simulink model "damiao"  (R2022b)
settings: Solver=VariableStepAuto  StartTime=0.0  StopTime=inf  RelTol=1e-3
libraries: simulink x4, RTBoxbasiclib x1, etargetslib x1
settings Model: Creator=admin  LastModifiedBy=admin

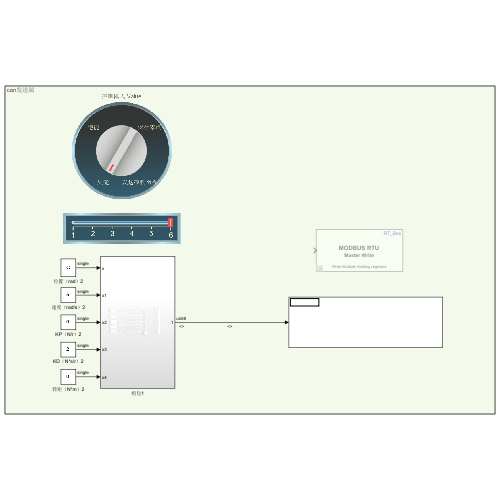
[thumbnail: Simulink's stored preview of the top-level diagram]
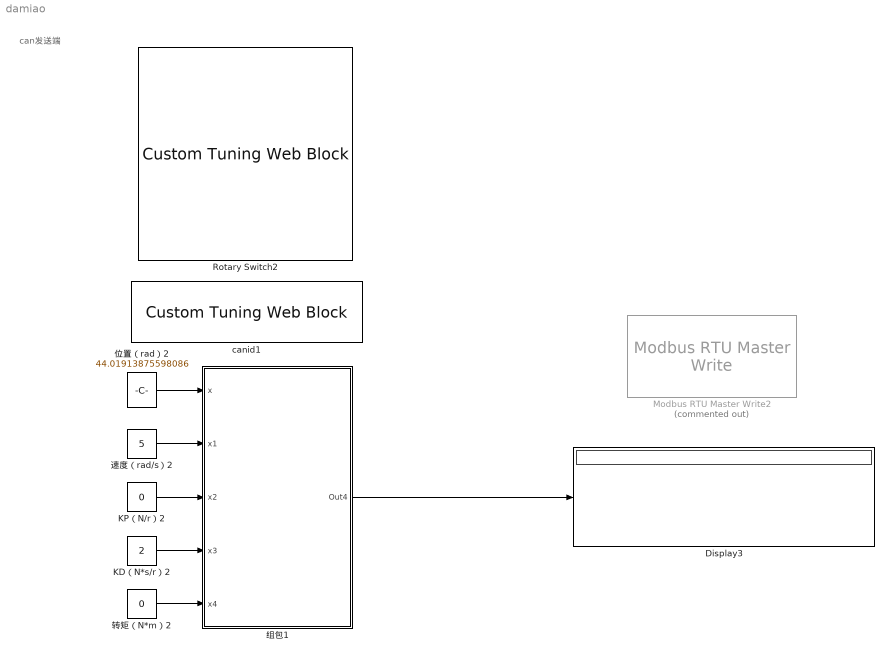
== system damiao ==
  note: can发送端
  Display3 : Display
      settings: Format=hex (Stored Integer)
  KD（N*s/r）2 : Constant  Value=2  OutDataTypeStr=single
  KP（N/r）2 : Constant  Value=0  OutDataTypeStr=single
  Modbus RTU Master Write2 : RTBoxbasiclib/Modbus RTU Master Write  Commented=on  Server_Port=/dev/ttyUSB0  Function=Write Multiple Holding registers  CoilAddress=0  HoldingRegisterAddress=0  numElements_coil=1  numElements_holdingReg=8  SampleTime=0.1  Slave_ID=1  Baudrate=1000  parity_=N  data_bit=8  stop_bit=1  responese_to_sec=0  responese_to_usec=0
      settings: SourceProductName=RT Box Simulink support
  Rotary Switch2 : CustomTuningWebBlock  ShowInitialText=on  Configuration="{\"type\":\"RotarySwitch\",\"settings\":{\"BindingType\":\"param\",\"backgroundColor\":[0,0,255,\"1\"],\"backgroundOffset\":1,\"fixedAspectRatio\":\"on\",\"image\":{\"size\":[150,150],\"src\":\"data:image/svg+xml;base64,PD94bWwgdmVyc2lvbj0iMS4wIiBlbmNvZGluZz0iVVRGLTgiIHN0YW5kYWxvbmU9Im5vIj8+CjwhLS0gR2VuZXJhdG9yOiBBZG9iZSBJbGx1c3RyYXRvciAxOS4yLjEsIFNWRyBFeHBvcnQgUGx1Zy1JbiAuIFNWRyBWZXJzaW9uOiA2LjAwIEJ1aWxkIDApICAtLT4KCjxzdmcKICAgeG1sbnM6ZGM9Imh0dHA6Ly9wdXJsLm9yZy9kYy9lbGVtZW50cy8xLjEvIgogICB4bWxuczpjYz0iaHR0cDovL2NyZWF0aXZlY29tbW9ucy5vcmcvbnMjIgogICB4bWxuczpyZGY9Imh0dHA6Ly93d3cudzMub3JnLzE5OTkvMDIvMjItcmRmLXN5bnRh ...(+9660 chars)\"},\"showBackgroundColor\":false,\"variant\":\"rotarySwitch\"},\"components\":[{\"name\":\"RotarySwitchComponent\",\"settings\":{\"arcAngle\":300,\"arcAngleOffset\":120,\"handle\":{\"size\":[150,150],\"src\":\"data:image/svg+xml;base64,PHN2ZyBpZD0iTGF5ZXJfMSIgZGF0YS1uYW1lPSJMYXllciAxIiB4bWxucz0iaHR0cDovL3d3dy53My5vcmcvMjAwMC9zdmciIHhtbG5zOnhsaW5rPSJodHRwOi8vd3d3LnczLm9yZy8xOTk5L3hsaW5rIiB2aWV3Qm94PSIwIDAgMTIxIDEyMSI+PGRlZnM+PHN0eWxlPi5jbHMtMXtmaWxsOnVybCgjbGluZWFyLWdyYWRpZW50KTt9LmNscy0yLC5jbHMtM3tmaWxsOiNkMWQxZDE7fS5jbHMtM3tzdHJva2U6I2I3YjdiNztzdHJva2UtbWl0ZXJsaW1pdDoxMDtzdHJva2Utd2lkdGg6MC4yNXB4O30uY2xzLTR7ZmlsbDojZjMwMDAwO30uY2xzLTV7ZmlsbDojZjIxNzY3O308L3N0eWxlPjxsaW5lYXJHcmFkaWVudCBpZD0ibGluZWFyLWdyYWRpZW50IiB4MT0iNjAuNSIgeTE9IjEyMC41IiB4Mj0iNjAuNSIgeTI9IjAuNSIgZ3JhZGllbnRVbml0cz0idXNlclNwYWNlT25Vc2UiPjxzdG9wIG9mZnNldD0iMCIgc3RvcC1jb2xvcj0iI2QxZDFkMSIvPjxzdG9wIG9mZnNldD0iMC4xIiBzdG9wLWNvbG9yPSIjY2VjZWNlIi8+PHN0b3Agb2Zmc2V0PSIwLjE5IiBzdG9wLWNvbG9yPSIjYzNjM2MzIi8+PHN0b3Agb2Zmc2V0PSIwLjI4IiBzdG9wLWNvbG9yPSIjYjFiMWIxIi8+PHN0b3Agb2Zmc2V0PSIwLjM2IiBzdG9wLWNvbG9yPSIjOTg5ODk4Ii8+PHN0b3Agb2Zmc2V0PSIwLjQ0IiBzdG9wLWNvbG9yPSIjNzg3ODc4Ii8+PHN0b3Agb2Zmc2V0PSIwLjQ2IiBzdG9wLWNvbG9yPSIjNmI2YjZiIi8+PHN0b3Agb2Zmc2V0PSIwLjU0IiBzdG9wLWNvbG9yPSIjNmI2YjZiIi8+PHN0b3Agb2Zmc2V0PSIwLjU2IiBzdG9wLWNvbG9yPSIjNzY3Njc2Ii8+PHN0b3Agb2Zmc2V0PSIwLjY0IiBzdG9wLWNvbG9yPSIjOTc5Nzk3Ii8+PHN0b3Agb2Zmc2V0PSIwLjcyIiBzdG9wLWNvbG9yPSIjYjBiMGIwIi8+PHN0b3Agb2Zmc2V0PSIwLjgxIiBzdG9wLWNvbG9yPSIjYzNjM2MzIi8+PHN0b3Agb2Zmc2V0PSIwLjkiIHN0b3AtY29sb3I9IiNjZGNkY2QiLz48c3RvcCBvZmZzZXQ9IjEiIHN0b3AtY29sb3I9IiNkMWQxZDEiLz48L2xpbmVhckdyYWRpZW50PjwvZGVmcz48Y2lyY2xlIGNsYXNzPSJjbHMtMSIgY3g9IjYwLjUiIGN5PSI2MC41IiByPSI2MCIvPjxwYXRoIGNsYXNzPSJjbHMtMiIgZD0iTTYwLjUsMUE1OS41LDU5LjUsMCwxLDEsMSw2MC41LDU5LjU3LDU5LjU3LDAsMCwxLDYwLjUsMW0wLTFBNjAuNSw2MC41LDAsMSwwLDEyMSw2MC41LDYwLjUsNjAuNSwwLDAsMCw2MC41LDBaIi8+PHJlY3QgY2xhc3M9ImNscy0zIiB4PSIwLjUiIHk9IjUxLjUiIHdpZHRoPSIxMjAiIGhlaWdodD0iMTgiIHJ4PSIzLjA0Ii8+PHJlY3QgY2xhc3M9ImNscy00IiB4PSI1Ljc1IiB5PSI1OC43NSIgd2lkdGg9IjE2IiBoZWlnaHQ9IjMiLz48cGF0aCBjbGFzcz0iY2xzLTUiIGQ9Ik0yMS4yNSw1OS4yNXYyaC0xNXYtMmgxNW0xLTFoLTE3djRoMTd2LTRaIi8+PC9zdmc+\"},\"handleOffset\":[0,0],\"handleOrientation\":180,\"handlePosition\":[0,0,1,1],\"handleSize\":{\"height\":0.5,\"width\":0.5},\"labelRadius\":0.36,\"position\":[0,0,1,1],\"states\":[{\"Label\":{\"color\":[0,0,0,1],\"icon\":{\"size\":[0,0],\"src\":[],\"srcOrientation\":\"Right\"},\"iconPlacement\":\"left\",\"opacity\":1,\"position\":[0.7345552884615385,0.6796274038461538],\"show\":true,\"text\":{\"content\":\"失能\",\"font\":\"Helvetica\",\"fontSize\":24}},\"Value\":0},{\"Label\":{\"color\":[0,0,0,1],\"icon\":{\"size\":[0,0],\"src\":[],\"srcOrientation\":\"Right\"},\"iconPlacement\":\"left\",\"opacity\":1,\"position\":[0.35757211538461536,0.7603966346153846],\"show\":true,\"text\":{\"content\":\"使能\",\"font\":\"Helvetica\",\"fontSize\":24}},\"Value\":1},{\"Label\":{\"color\":[0,0,0,1],\"icon\":{\"size\":[0,0],\"src\":[],\"srcOrientation\":\"Right\"},\"iconPlacement\":\"left\",\"opacity\":1,\"position\":[0.09603365384615385,0.46033653846153844],\"show\":true,\"text\":{\"content\":\"保存零点\",\"font\":\"Helvetica\",\"fontSize\":24}},\"Value\":2},{\"Label\":{\"color\":[0,0,0,1],\"icon\":{\"size\":[0,0],\"src\":[],\"srcOrientation\":\"Right\"},\"iconPlacement\":\"left\",\"opacity\":1,\"position\":[0.36532451923076925,0.1180889423076923],\"show\":true,\"text\":{\"content\":\"发送控制命令\",\"font\":\"Helvetica\",\"fontSize\":24}},\"Value\":3}],\"tickRadius\":0.32}},{\"name\":\"BackgroundImageComponent\",\"settings\":{\"image\":{\"size\":[155,150],\"src\":\"data:image/svg+xml;base64,PD94bWwgdmVyc2lvbj0iMS4wIiBlbmNvZGluZz0idXRmLTgiPz4NCjwhLS0gR2VuZXJhdG9yOiBBZG9iZSBJbGx1c3RyYXRvciAyNS4wLjAsIFNWRyBFeHBvcnQgUGx1Zy1JbiAuIFNWRyBWZXJzaW9uOiA2LjAwIEJ1aWxkIDApICAtLT4NCjxzdmcgdmVyc2lvbj0iMS4xIg0KCSBpZD0iTGF5ZXJfMl8xXyIgeG1sbnM6Y2M9Imh0dHA6Ly9jcmVhdGl2ZWNvbW1vbnMub3JnL25zIyIgeG1sbnM6ZGM9Imh0dHA6Ly9wdXJsLm9yZy9kYy9lbGVtZW50cy8xLjEvIiB4bWxuczppbmtzY2FwZT0iaHR0cDovL3d3dy5pbmtzY2FwZS5vcmcv ...(+4184 chars)\",\"srcOrientation\":\"Right\"},\"position\":[0,0,1,1],\"scaleMode\":\"0\"}},{\"name\":\"ForegroundImageComponent\",\"settings\":{\"image\":{\"size\":[0,0],\"src\":\"default\",\"srcOrientation\":[]},\"isForeground\":1,\"position\":[0,0,1,1],\"scaleMode\":\"0\"}}]}"
  canid1 : CustomTuningWebBlock  LabelPosition=Hide  ShowInitialText=on  Configuration="{\"type\":\"LinearGauge\",\"settings\":{\"BindingType\":\"param\",\"aspectRatio\":3.7777777777777777,\"backgroundColor\":[0,0,0,\"1\"],\"backgroundOffset\":0,\"backgroundOpacity\":1,\"fixedAspectRatio\":\"on\",\"foregroundColor\":[252,252,196],\"orientation\":\"horizontal\",\"showBackgroundColor\":false,\"value\":0},\"components\":[{\"name\":\"LinearScaleComponent\",\"settings\":{\"bounds\":{\"max\":6,\"min\":1,\"tickInterval\":1},\"internalTickHeightScaleFactor\":0.5,\"labelColor\":[255,255,200],\"labelFont\":{\"font\":\"Arial\",\"fontSize\":12},\"labelOffset\":0.05,\"labelTransparency\":1,\"needleImage\":{\"size\":[596,842],\"src\":\"data:image/svg+xml;base64,PD94bWwgdmVyc2lvbj0iMS4wIiBlbmNvZGluZz0idXRmLTgiPz4NCjwhLS0gR2VuZXJhdG9yOiBBZG9iZSBJbGx1c3RyYXRvciAyNS4wLjAsIFNWRyBFeHBvcnQgUGx1Zy1JbiAuIFNWRyBWZXJzaW9uOiA2LjAwIEJ1aWxkIDApICAtLT4NCjxzdmcgdmVyc2lvbj0iMS4xIg0KCSBpZD0ic3ZnOCIgeG1sbnM6Y2M9Imh0dHA6Ly9jcmVhdGl2ZWNvbW1vbnMub3JnL25zIyIgeG1sbnM6ZGM9Imh0dHA6Ly9wdXJsLm9yZy9kYy9lbGVtZW50cy8xLjEvIiB4bWxuczppbmtzY2FwZT0iaHR0cDovL3d3dy5pbmtzY2FwZS5vcmcvbmFtZXNw ...(+2420 chars)\",\"srcOrientation\":\"Right\"},\"needleOffset\":[-0.8044596912521441,-0.0642123287671233],\"needleSize\":{\"height\":0.4337797619047619,\"width\":0.07668067226890757},\"position\":[0.2829861111111111,0.04398634453781513,0.9196428571428571,0.6088789682539683],\"referencePoint\":\"auto\",\"scaleColors\":[],\"scaleColorsSize\":0.2,\"scaleDirection\":\"LR\",\"showLabels\":1,\"showMinorTicks\":0,\"showSpanLine\":1,\"showTicks\":1,\"tickColor\":[252,252,197],\"tickTransparency\":1,\"valueBarColor\":[0,114,189],\"valueBarOffset\":-0.27,\"valueBarSize\":0.1,\"valueBarTransparency\":1}},{\"name\":\"BackgroundImageComponent\",\"settings\":{\"image\":{\"size\":[380,101],\"src\":\"data:image/svg+xml;base64,PHN2ZyB4bWxucz0iaHR0cDovL3d3dy53My5vcmcvMjAwMC9zdmciIHhtbG5zOnhsaW5rPSJodHRwOi8vd3d3LnczLm9yZy8xOTk5L3hsaW5rIiB2aWV3Qm94PSIwIDAgMzgwIDEwMSI+PGRlZnM+PHN0eWxlPi5jbHMtMXtmaWxsOiMwMDJiNDI7fS5jbHMtMntmaWxsOiM0MjcwODI7fS5jbHMtM3tmaWxsOnVybCgjcmFkaWFsLWdyYWRpZW50KTt9LmNscy00e2ZpbGw6I2M4YzhjODtzdHJva2U6IzAwMDt9PC9zdHlsZT48cmFkaWFsR3JhZGllbnQgaWQ9InJhZGlhbC1ncmFkaWVudCIgY3g9IjE5MCIgY3k9IjUwLjUiIHI9IjI2OS4yMSIgZ3JhZGllbnRVbml0cz0idXNlclNwYWNlT25Vc2UiPjxzdG9wIG9mZnNldD0iMC4wMSIgc3RvcC1jb2xvcj0iIzNlNGY1OCIvPjxzdG9wIG9mZnNldD0iMC4wNiIgc3RvcC1jb2xvcj0iIzQ0NTc2MSIvPjxzdG9wIG9mZnNldD0iMC4xNSIgc3RvcC1jb2xvcj0iIzU1NmE3NiIvPjxzdG9wIG9mZnNldD0iMC4yNSIgc3RvcC1jb2xvcj0iIzZkODg5NSIvPjxzdG9wIG9mZnNldD0iMC4zOCIgc3RvcC1jb2xvcj0iIzhmYjJjMyIvPjxzdG9wIG9mZnNldD0iMC41MiIgc3RvcC1jb2xvcj0iI2I2ZTRmYSIvPjxzdG9wIG9mZnNldD0iMSIgc3RvcC1jb2xvcj0iIzE1NDY1NyIvPjwvcmFkaWFsR3JhZGllbnQ+PC9kZWZzPjxnIGlkPSJmcmFtZSI+PGcgaWQ9IkxheWVyXzIiIGRhdGEtbmFtZT0iTGF5ZXIgMiI+PGcgaWQ9IkxheWVyXzEtMiIgZGF0YS1uYW1lPSJMYXllciAxLTIiPjxyZWN0IGlkPSJyZWN0MTAzNiIgY2xhc3M9ImNscy0xIiB4PSIxMSIgeT0iMTEiIHdpZHRoPSIzNTgiIGhlaWdodD0iNzkiLz48cGF0aCBpZD0icGF0aDEwMzgiIGNsYXNzPSJjbHMtMiIgZD0iTTgsOFY5M0gzNzJWOFpNMzY5LDkwSDExVjExSDM2OVoiLz48cGF0aCBpZD0icGF0aDEwNDAiIGNsYXNzPSJjbHMtMyIgZD0iTTAsMFYxMDFIMzgwVjBaTTM3Miw5M0g4VjhIMzcyWiIvPjwvZz48L2c+PC9nPjxnIGlkPSJ0cmFjayI+PHBhdGggaWQ9InJlY3QxNjExIiBjbGFzcz0iY2xzLTQiIGQ9Ik0zMy4zNywyNi41OUgzNDYuNjNjNCwwLDcuMjUsMi42LDcuMjUsNS44MWgwYzAsMy4yMS0zLjI1LDUuODItNy4yNSw1LjgySDMzLjM3Yy00LDAtNy4yNS0yLjYxLTcuMjUtNS44MmgwQzI2LjEyLDI5LjE5LDI5LjM3LDI2LjU5LDMzLjM3LDI2LjU5WiIvPjwvZz48L3N2Zz4=\",\"srcOrientation\":\"horizontal\"},\"position\":[0,0,1,1],\"scaleMode\":\"0\"}},{\"name\":\"ForegroundImageComponent\",\"settings\":{\"image\":{\"size\":[0,0],\"src\":\"default\",\"srcOrientation\":[]},\"isForeground\":1,\"position\":[0,0,1,1],\"scaleMode\":\"0\"}}]}"
  位置（rad）2 : Constant  Value=44.01913875598086  OutDataTypeStr=single
  组包1 : Subsystem
  转矩（N*m）2 : Constant  Value=0  OutDataTypeStr=single
  速度（rad/s）2 : Constant  Value=5  OutDataTypeStr=single
  wires:
  KP（N/r）2/1 -> 组包1/3(x2)
  组包1/1(Out4) -> Display3/1
  KD（N*s/r）2/1 -> 组包1/4(x3)
  转矩（N*m）2/1 -> 组包1/5(x4)
  速度（rad/s）2/1 -> 组包1/2(x1)
  位置（rad）2/1 -> 组包1/1(x)

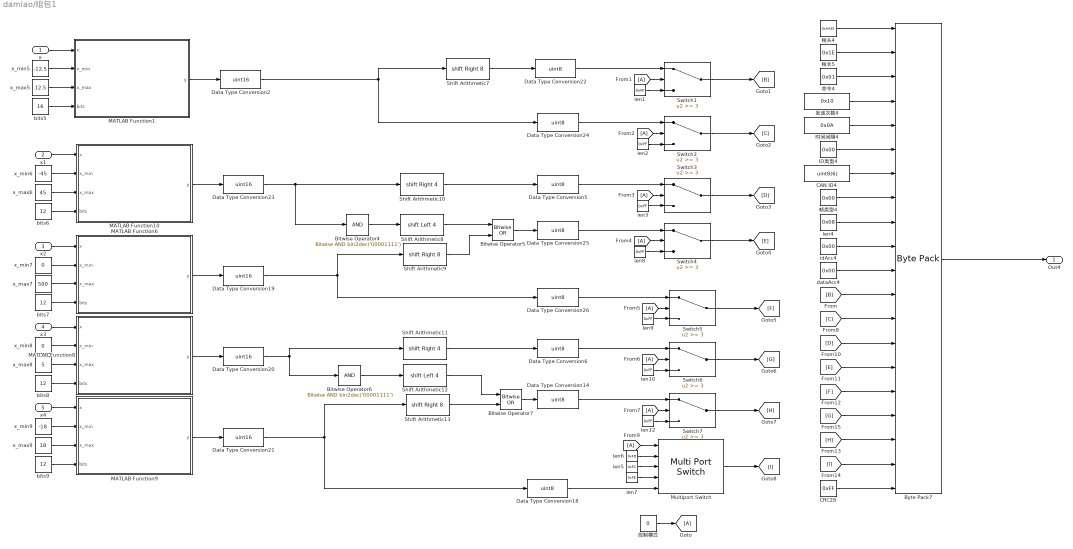
== system damiao/组包1 ==
  x : Inport
  x1 : Inport  Port=2
  x2 : Inport  Port=3
  x3 : Inport  Port=4
  x4 : Inport  Port=5
  Bitwise Operator4 : simulink/Logic and Bit Operations/Bitwise Operator  logicop=AND  UseBitMask=on  BitMask=bin2dec('00001111')  BitMaskRealWorld=Stored Integer
  Bitwise Operator5 : simulink/Logic and Bit Operations/Bitwise Operator  logicop=OR  UseBitMask=off  NumInputPorts=2  BitMask=bin2dec('00001000')  BitMaskRealWorld=Stored Integer
  Bitwise Operator6 : simulink/Logic and Bit Operations/Bitwise Operator  logicop=AND  UseBitMask=on  BitMask=bin2dec('00001111')  BitMaskRealWorld=Stored Integer
  Bitwise Operator7 : simulink/Logic and Bit Operations/Bitwise Operator  logicop=OR  UseBitMask=off  NumInputPorts=2  BitMask=bin2dec('00001000')  BitMaskRealWorld=Stored Integer
  Byte Pack7 : etargetslib/Byte Pack  datatypes={'uint16','uint8','uint8','uint32','uint32','uint8','uint32','uint8','uint8','uint8','uint8','uint8','uint8','uint8','uint8','uint8','uint8','uint8','uint8','uint8'}  byteAlign=1
  CAN ID4 : Constant  Value=uint8(6)  OutDataTypeStr=uint32
  CRC28 : Constant  Value=0xFF  OutDataTypeStr=uint8
  Data Type Conversion{5..6,14,18,22,24..26} (8 alike) : DataTypeConversion  OutDataTypeStr=uint8  SaturateOnIntegerOverflow=off  RndMeth=Floor
  Data Type Conversion{2,19..21,23} (5 alike) : DataTypeConversion  OutDataTypeStr=uint16  SaturateOnIntegerOverflow=off  RndMeth=Floor
  From{1..7,9} (8 alike) : From
  Goto : Goto
  ID类型4 : Constant  Value=0x00  OutDataTypeStr=uint8
  MATLAB Function1 : MATLAB Function  TreatAsAtomicUnit=on
  MATLAB Function10 : MATLAB Function  TreatAsAtomicUnit=on
  MATLAB Function6 : MATLAB Function  TreatAsAtomicUnit=on
  MATLAB Function8 : MATLAB Function  TreatAsAtomicUnit=on
  MATLAB Function9 : MATLAB Function  TreatAsAtomicUnit=on
  Multiport Switch : MultiPortSwitch  DataPortOrder=Zero-based contiguous  Inputs=4  zeroidx=on  SaturateOnIntegerOverflow=off  InputSameDT=off
  Shift Arithmetic10 : ArithShift  BitShiftNumber=4  BitShiftDirection=Right
  Shift Arithmetic11 : ArithShift  BitShiftNumber=4  BitShiftDirection=Right
  Shift Arithmetic12 : ArithShift  BitShiftNumber=4  BitShiftDirection=Left
  Shift Arithmetic13 : ArithShift  BitShiftNumber=8  BitShiftDirection=Right
  Shift Arithmetic7 : ArithShift  BitShiftNumber=8  BitShiftDirection=Right
  Shift Arithmetic8 : ArithShift  BitShiftNumber=4  BitShiftDirection=Left
  Shift Arithmetic9 : ArithShift  BitShiftNumber=8  BitShiftDirection=Right
  Switch{1..7} (7 alike) : Switch  Threshold=3  SaturateOnIntegerOverflow=off  InputSameDT=off
  bits5 : Constant  Value=16  OutDataTypeStr=uint16
  bits{6..9} (4 alike) : Constant  Value=12  OutDataTypeStr=uint16
  dataAcc4 : Constant  Value=0x00  OutDataTypeStr=uint8
  idAcc4 : Constant  Value=0x00  OutDataTypeStr=uint8
  len{1..3,8..10,12} (7 alike) : Constant  Value=0xFF  OutDataTypeStr=uint8
  len4 : Constant  Value=0x08  OutDataTypeStr=uint8
  len5 : Constant  Value=0xFC  OutDataTypeStr=uint8
  len6 : Constant  Value=0xFD  OutDataTypeStr=uint8
  len7 : Constant  Value=0xFE  OutDataTypeStr=uint8
  x_max5 : Constant  Value=12.5  OutDataTypeStr=single
  x_max6 : Constant  Value=45  OutDataTypeStr=single
  x_max7 : Constant  Value=500  OutDataTypeStr=single
  x_max8 : Constant  Value=5  OutDataTypeStr=single
  x_max9 : Constant  Value=18  OutDataTypeStr=single
  x_min5 : Constant  Value=-12.5  OutDataTypeStr=single
  x_min6 : Constant  Value=-45  OutDataTypeStr=single
  x_min7 : Constant  Value=0  OutDataTypeStr=single
  x_min8 : Constant  Value=0  OutDataTypeStr=single
  x_min9 : Constant  Value=-18  OutDataTypeStr=single
  发送次数4 : Constant  Value=0x10  OutDataTypeStr=uint32
  命令4 : Constant  Value=0x01  OutDataTypeStr=uint8
  帧头4 : Constant  Value=0xAA55  OutDataTypeStr=uint16
  帧类型4 : Constant  Value=0x00  OutDataTypeStr=uint8
  帧长5 : Constant  Value=0x1E  OutDataTypeStr=uint8
  控制模式 : Constant  Value=0  OutDataTypeStr=int8
  时间间隔4 : Constant  Value=0x0A  OutDataTypeStr=uint32
  Out4 : Outport
  wires:
  MATLAB Function10/1(y) -> Data Type Conversion23/1
  Data Type Conversion23/1 -> Shift Arithmetic10/1, Bitwise Operator4/1
  MATLAB Function6/1(y) -> Data Type Conversion19/1
  Bitwise Operator5/1 -> Data Type Conversion25/1
  Bitwise Operator6/1 -> Shift Arithmetic12/1
  发送次数4/1 -> Byte Pack7/4
  Data Type Conversion2/1 -> Data Type Conversion24/1, Shift Arithmetic7/1
  bits5/1 -> MATLAB Function1/4(bits)
  MATLAB Function9/1(y) -> Data Type Conversion21/1
  Shift Arithmetic10/1 -> Data Type Conversion5/1
  bits8/1 -> MATLAB Function8/4(bits)
  len4/1 -> Byte Pack7/9
  x_max8/1 -> MATLAB Function8/3(x_max)
  idAcc4/1 -> Byte Pack7/10
  Shift Arithmetic13/1 -> Bitwise Operator7/2
  x_max7/1 -> MATLAB Function6/3(x_max)
  Bitwise Operator4/1 -> Shift Arithmetic8/1
  x_min7/1 -> MATLAB Function6/2(x_min)
  x_max5/1 -> MATLAB Function1/3(x_max)
  Bitwise Operator7/1 -> Data Type Conversion14/1
  Data Type Conversion19/1 -> Data Type Conversion26/1, Shift Arithmetic9/1
  Shift Arithmetic12/1 -> Bitwise Operator7/1
  x2/1 -> MATLAB Function6/1(x)
  时间间隔4/1 -> Byte Pack7/5
  bits9/1 -> MATLAB Function9/4(bits)
  MATLAB Function8/1(y) -> Data Type Conversion20/1
  Shift Arithmetic8/1 -> Bitwise Operator5/1
  Shift Arithmetic9/1 -> Bitwise Operator5/2
  bits7/1 -> MATLAB Function6/4(bits)
  x_min9/1 -> MATLAB Function9/2(x_min)
  帧类型4/1 -> Byte Pack7/8
  dataAcc4/1 -> Byte Pack7/11
  x_max6/1 -> MATLAB Function10/3(x_max)
  Shift Arithmetic7/1 -> Data Type Conversion22/1
  bits6/1 -> MATLAB Function10/4(bits)
  Byte Pack7/1 -> Out4/1
  x_min8/1 -> MATLAB Function8/2(x_min)
  x_min6/1 -> MATLAB Function10/2(x_min)
  Data Type Conversion20/1 -> Shift Arithmetic11/1, Bitwise Operator6/1
  x_min5/1 -> MATLAB Function1/2(x_min)
  Data Type Conversion21/1 -> Shift Arithmetic13/1, Data Type Conversion18/1
  CAN ID4/1 -> Byte Pack7/7
  MATLAB Function1/1(y) -> Data Type Conversion2/1
  ID类型4/1 -> Byte Pack7/6
  Shift Arithmetic11/1 -> Data Type Conversion6/1
  x_max9/1 -> MATLAB Function9/3(x_max)
  命令4/1 -> Byte Pack7/3
  帧头4/1 -> Byte Pack7/1
  CRC28/1 -> Byte Pack7/20
  帧长5/1 -> Byte Pack7/2
  x/1 -> MATLAB Function1/1(x)
  x1/1 -> MATLAB Function10/1(x)
  x4/1 -> MATLAB Function9/1(x)
  x3/1 -> MATLAB Function8/1(x)
  len1/1 -> Switch1/3
  From1/1 -> Switch1/2
  控制模式/1 -> Goto/1
  len2/1 -> Switch2/3
  From2/1 -> Switch2/2
  From3/1 -> Switch3/2
  len3/1 -> Switch3/3
  len10/1 -> Switch6/3
  len9/1 -> Switch5/3
  len8/1 -> Switch4/3
  From4/1 -> Switch4/2
  From6/1 -> Switch6/2
  From5/1 -> Switch5/2
  len12/1 -> Switch7/3
  From7/1 -> Switch7/2
  Data Type Conversion22/1 -> Switch1/1
  Data Type Conversion24/1 -> Switch2/1
  Data Type Conversion5/1 -> Switch3/1
  Data Type Conversion25/1 -> Switch4/1
  Data Type Conversion26/1 -> Switch5/1
  Data Type Conversion6/1 -> Switch6/1
  Data Type Conversion14/1 -> Switch7/1
  Data Type Conversion18/1 -> Multiport Switch/5
  len6/1 -> Multiport Switch/2
  len5/1 -> Multiport Switch/3
  From9/1 -> Multiport Switch/1
  len7/1 -> Multiport Switch/4
  Switch1/1 -> [B]
  [B] -> Byte Pack7/12
  Switch2/1 -> [C]
  [C] -> Byte Pack7/13
  Switch3/1 -> [D]
  Switch4/1 -> [E]
  Switch5/1 -> [F]
  Switch7/1 -> [H]
  Switch6/1 -> [G]
  Multiport Switch/1 -> [I]
  [D] -> Byte Pack7/14
  [E] -> Byte Pack7/15
  [F] -> Byte Pack7/16
  [G] -> Byte Pack7/17
  [H] -> Byte Pack7/18
  [I] -> Byte Pack7/19

== matlab function damiao/组包1/MATLAB Function1 ==
  data: x input; y output; x_min input; x_max input; bits input
function y = float_to_uint(x, x_min, x_max, bits)
% Converts a float to an unsigned int, given range and number of bits

% 简单的参数检查（无字符串信息）
if ~(isa(x, 'single') || isa(x, 'double'))
    y = int32(0);  % 返回 0 表示错误
    return;
end

if ~(isa(x_min, 'single') || isa(x_min, 'double')) || ...
   ~(isa(x_max, 'single') || isa(x_max, 'double')) || ...
    ~isscalar(bits) || bits <= 0
    y = int32(0);  % 返回 0 表示错误
    return;
end

% 计算范围和偏移量
span = single(x_max - x_min);
offset = single(x_min);

% 转换
y = int32((single(x) - offset) * single((2^bits - 1)) / span);
end

== matlab function damiao/组包1/MATLAB Function10 ==
  data: x input; y output; x_min input; x_max input; bits input
function y = float_to_uint(x, x_min, x_max, bits)
% Converts a float to an unsigned int, given range and number of bits

% 简单的参数检查（无字符串信息）
if ~(isa(x, 'single') || isa(x, 'double'))
    y = int32(0);  % 返回 0 表示错误
    return;
end

if ~(isa(x_min, 'single') || isa(x_min, 'double')) || ...
   ~(isa(x_max, 'single') || isa(x_max, 'double')) || ...
    ~isscalar(bits) || bits <= 0
    y = int32(0);  % 返回 0 表示错误
    return;
end

% 计算范围和偏移量
span = single(x_max - x_min);
offset = single(x_min);

% 转换
y = int32((single(x) - offset) * single((2^bits - 1)) / span);
end

== matlab function damiao/组包1/MATLAB Function6 ==
  data: x input; y output; x_min input; x_max input; bits input
function y = float_to_uint(x, x_min, x_max, bits)
% Converts a float to an unsigned int, given range and number of bits

% 简单的参数检查（无字符串信息）
if ~(isa(x, 'single') || isa(x, 'double'))
    y = int32(0);  % 返回 0 表示错误
    return;
end

if ~(isa(x_min, 'single') || isa(x_min, 'double')) || ...
   ~(isa(x_max, 'single') || isa(x_max, 'double')) || ...
    ~isscalar(bits) || bits <= 0
    y = int32(0);  % 返回 0 表示错误
    return;
end

% 计算范围和偏移量
span = single(x_max - x_min);
offset = single(x_min);

% 转换
y = int32((single(x) - offset) * single((2^bits - 1)) / span);
end

== matlab function damiao/组包1/MATLAB Function8 ==
  data: x input; y output; x_min input; x_max input; bits input
function y = float_to_uint(x, x_min, x_max, bits)
% Converts a float to an unsigned int, given range and number of bits

% 简单的参数检查（无字符串信息）
if ~(isa(x, 'single') || isa(x, 'double'))
    y = int32(0);  % 返回 0 表示错误
    return;
end

if ~(isa(x_min, 'single') || isa(x_min, 'double')) || ...
   ~(isa(x_max, 'single') || isa(x_max, 'double')) || ...
    ~isscalar(bits) || bits <= 0
    y = int32(0);  % 返回 0 表示错误
    return;
end

% 计算范围和偏移量
span = single(x_max - x_min);
offset = single(x_min);

% 转换
y = int32((single(x) - offset) * single((2^bits - 1)) / span);
end

== matlab function damiao/组包1/MATLAB Function9 ==
  data: x input; y output; x_min input; x_max input; bits input
function y = float_to_uint(x, x_min, x_max, bits)
% Converts a float to an unsigned int, given range and number of bits

% 简单的参数检查（无字符串信息）
if ~(isa(x, 'single') || isa(x, 'double'))
    y = int32(0);  % 返回 0 表示错误
    return;
end

if ~(isa(x_min, 'single') || isa(x_min, 'double')) || ...
   ~(isa(x_max, 'single') || isa(x_max, 'double')) || ...
    ~isscalar(bits) || bits <= 0
    y = int32(0);  % 返回 0 表示错误
    return;
end

% 计算范围和偏移量
span = single(x_max - x_min);
offset = single(x_min);

% 转换
y = int32((single(x) - offset) * single((2^bits - 1)) / span);
end
